simulink model "Hybrid2_article_SVC_stage1"  (R2025a)
settings: Solver=FixedStepAuto  StartTime=0.0  StopTime=0.2  FixedStep=Ts  RelTol=1e-3
undefined symbols (not defined in the file or in its folder): closedLoop, controller, D1, D11, Delta, DiscIntNeverNeededParam, find_system, grid, level, protection, sensor, solarPanel, solarPlant, Ts
libraries: powerlib_extras x38, nesl_utility x29, spsSampleandHoldLib x24, spsThyristorLib x24, spsSeriesRLCBranchLib x23, simulink x22, fl_lib x18, ee_lib x12, spsEdgeDetectorLib x12, spsParallelRLCBranchLib x10, spsThreePhaseVIMeasurementLib x9, simulink_extras x8
(part 6 of 8)

== system Hybrid2_article_SVC_stage1/Distribution Statcom1/D_statcom_avg Controller/Controller (sample time=Ts*32)/Current Regulator ==
  note: =================
  note: Current Regulators
  IdIq : Inport  PortDimensions=2
  IdIq_Ref : Inport  Port=2  PortDimensions=2
  Demux : Demux  Outputs=2
      settings: DisplayOption=none
  Demux1 : Demux  Outputs=2
      settings: DisplayOption=none
  Discrete PID Controller1 : slpidlib/PID Controller  Controller=PI  Form=Parallel  TimeDomain=Discrete-time  UseExternalTs=off  SampleTime=Ts  IntegratorMethod=Forward Euler  FilterMethod=Forward Euler  ControllerParametersSource=internal  P=Kp  I=Ki  UseKiTs=off  D=0  UseExternalDerivativeSource=off  N=100  UseFilter=on  TunerSelectOption=Transfer Function Based (PID Tuner App)  InitialConditionSource=internal  InitialConditionForIntegrator=0  InitialConditionForFilter=0  DifferentiatorICPrevScaledInput=0  ExternalReset=none  TrackingMode=off  Kt=1  LimitOutput=on  SatLimitsSource=internal  UpperSaturationLimit=1  LowerSaturationLimit=-1  LinearizeAsGain=off  AntiWindupMode=clamping  Kb=1  LimitIntegrator=off  UpperIntegratorSaturationLimit=inf  LowerIntegratorSaturationLimit=-inf  POutMin=[]  POutMax=[]  IOutMin=[]  IOutMax=[]  DOutMin=[]  DOutMax=[]  NOutMin=[]  NOutMax=[]  SumOutMin=[]  SumOutMax=[]  SaturationOutMin=[]  SaturationOutMax=[]  PParamMin=[]  PParamMax=[]  IParamMin=[]  IParamMax=[]  DParamMin=[]  DParamMax=[]  NParamMin=[]  NParamMax=[]  KbParamMin=[]  KbParamMax=[]  KtParamMin=[]  KtParamMax=[]  KbOutMin=[]  KbOutMax=[]  KtOutMin=[]  KtOutMax=[]  IntegratorOutMin=[]  IntegratorOutMax=[]  FilterOutMin=[]  FilterOutMax=[]  SumI1OutMin=[]  SumI1OutMax=[]  SumI2OutMin=[]  SumI2OutMax=[]  SumI3OutMin=[]  SumI3OutMax=[]  SumI4OutMin=[]  SumI4OutMax=[]  SumDOutMin=[]  SumDOutMax=[]  DifferentiatorOutMin=[]  DifferentiatorOutMax=[]  FilterDiffOutCoefMin=[]  FilterDiffOutCoefMax=[]  ReciprocalOutMin=[]  ReciprocalOutMax=[]  SumDenOutMin=[]  SumDenOutMax=[]  SumNumOutMin=[]  SumNumOutMax=[]  DivideOutMin=[]  DivideOutMax=[]  UdiffTsProdOutMin=[]  UdiffTsProdOutMax=[]  NTsProdOutMin=[]  NTsProdOutMax=[]  UintegralTsProdOutMin=[]  UintegralTsProdOutMax=[]  UngainTsProdOutMin=[]  UngainTsProdOutMax=[]  ClampingZeroOutDataTypeStr=Inherit: Inherit via back propagation  ClampingZeroOutMin=[]  ClampingZeroOutMax=[]  FilterDenConstantOutDataTypeStr=Inherit: Inherit via back propagation  FilterDenConstantOutMin=[]  FilterDenConstantOutMax=[]  PCopyOutDataTypeStr=Inherit: Inherit via back propagation  PCopyOutMin=[]  PCopyOutMax=[]  NCopyOutDataTypeStr=Inherit: Inherit via back propagation  NCopyOutMin=[]  NCopyOutMax=[]  IntegratorContinuousStateAttributes=''  IntegratorStateMustResolveToSignalObject=off  IntegratorRTWStateStorageClass=Auto  FilterContinuousStateAttributes=''  FilterStateMustResolveToSignalObject=off  FilterRTWStateStorageClass=Auto  ParallelPVariant=InternalParameters  IdealPVariant=Disabled  IVariant=InternalParameters  DVariant=Disabled  IntegratorVariant=Discrete  SatVariant=Enabled  AWVariant=DiscClampingParallel  PCopyVariant=Disabled  TRVariant=Disabled  FdbkBlocksVariant=Forward  IdealPFdbkVariant=Disabled  SatFdbkVariant=Disabled  DerivativeFilterVariant=Disabled  NVariant=Disabled  NCopyVariant=Disabled_SignalSpec  FilterICVariant=Disabled  IntegratorICVariant=InternalICs  ExternalResetVariant=Disabled  TRSumVariant=Passthrough  SumFdbkVariant=Disabled  SumVariant=Sum_PI  TsampFilterVariant=InternalTs  TsampNgainVariant=Passthrough  TsampIntegralVariant=Disabled_SignalSpec  ExternalSaturationOutDataTypeStr=Inherit: Same as second input  DerivativeSourceVariant=Disabled  PreIntVariant=InternalPreInt
      settings: AttributesFormatString=P = %<P>\nI = %<I>
  Discrete PID Controller2 : slpidlib/PID Controller  Controller=PI  Form=Parallel  TimeDomain=Discrete-time  UseExternalTs=off  SampleTime=Ts  IntegratorMethod=Forward Euler  FilterMethod=Forward Euler  ControllerParametersSource=internal  P=Kp  I=Ki  UseKiTs=off  D=0  UseExternalDerivativeSource=off  N=100  UseFilter=on  TunerSelectOption=Transfer Function Based (PID Tuner App)  InitialConditionSource=internal  InitialConditionForIntegrator=0  InitialConditionForFilter=0  DifferentiatorICPrevScaledInput=0  ExternalReset=none  TrackingMode=off  Kt=1  LimitOutput=on  SatLimitsSource=internal  UpperSaturationLimit=1  LowerSaturationLimit=-1  LinearizeAsGain=off  AntiWindupMode=clamping  Kb=1  LimitIntegrator=off  UpperIntegratorSaturationLimit=inf  LowerIntegratorSaturationLimit=-inf  POutMin=[]  POutMax=[]  IOutMin=[]  IOutMax=[]  DOutMin=[]  DOutMax=[]  NOutMin=[]  NOutMax=[]  SumOutMin=[]  SumOutMax=[]  SaturationOutMin=[]  SaturationOutMax=[]  PParamMin=[]  PParamMax=[]  IParamMin=[]  IParamMax=[]  DParamMin=[]  DParamMax=[]  NParamMin=[]  NParamMax=[]  KbParamMin=[]  KbParamMax=[]  KtParamMin=[]  KtParamMax=[]  KbOutMin=[]  KbOutMax=[]  KtOutMin=[]  KtOutMax=[]  IntegratorOutMin=[]  IntegratorOutMax=[]  FilterOutMin=[]  FilterOutMax=[]  SumI1OutMin=[]  SumI1OutMax=[]  SumI2OutMin=[]  SumI2OutMax=[]  SumI3OutMin=[]  SumI3OutMax=[]  SumI4OutMin=[]  SumI4OutMax=[]  SumDOutMin=[]  SumDOutMax=[]  DifferentiatorOutMin=[]  DifferentiatorOutMax=[]  FilterDiffOutCoefMin=[]  FilterDiffOutCoefMax=[]  ReciprocalOutMin=[]  ReciprocalOutMax=[]  SumDenOutMin=[]  SumDenOutMax=[]  SumNumOutMin=[]  SumNumOutMax=[]  DivideOutMin=[]  DivideOutMax=[]  UdiffTsProdOutMin=[]  UdiffTsProdOutMax=[]  NTsProdOutMin=[]  NTsProdOutMax=[]  UintegralTsProdOutMin=[]  UintegralTsProdOutMax=[]  UngainTsProdOutMin=[]  UngainTsProdOutMax=[]  ClampingZeroOutDataTypeStr=Inherit: Inherit via back propagation  ClampingZeroOutMin=[]  ClampingZeroOutMax=[]  FilterDenConstantOutDataTypeStr=Inherit: Inherit via back propagation  FilterDenConstantOutMin=[]  FilterDenConstantOutMax=[]  PCopyOutDataTypeStr=Inherit: Inherit via back propagation  PCopyOutMin=[]  PCopyOutMax=[]  NCopyOutDataTypeStr=Inherit: Inherit via back propagation  NCopyOutMin=[]  NCopyOutMax=[]  IntegratorContinuousStateAttributes=''  IntegratorStateMustResolveToSignalObject=off  IntegratorRTWStateStorageClass=Auto  FilterContinuousStateAttributes=''  FilterStateMustResolveToSignalObject=off  FilterRTWStateStorageClass=Auto  ParallelPVariant=InternalParameters  IdealPVariant=Disabled  IVariant=InternalParameters  DVariant=Disabled  IntegratorVariant=Discrete  SatVariant=Enabled  AWVariant=DiscClampingParallel  PCopyVariant=Disabled  TRVariant=Disabled  FdbkBlocksVariant=Forward  IdealPFdbkVariant=Disabled  SatFdbkVariant=Disabled  DerivativeFilterVariant=Disabled  NVariant=Disabled  NCopyVariant=Disabled_SignalSpec  FilterICVariant=Disabled  IntegratorICVariant=InternalICs  ExternalResetVariant=Disabled  TRSumVariant=Passthrough  SumFdbkVariant=Disabled  SumVariant=Sum_PI  TsampFilterVariant=InternalTs  TsampNgainVariant=Passthrough  TsampIntegralVariant=Disabled_SignalSpec  ExternalSaturationOutDataTypeStr=Inherit: Same as second input  DerivativeSourceVariant=Disabled  PreIntVariant=InternalPreInt
      settings: AttributesFormatString=P = %<P>\nI = %<I>
  Mux : Mux  Inputs=2
  Rate Limiter : RateLimiter  RisingSlewLimit=240  FallingSlewLimit=-240  SampleTimeMode=inherited
      settings: AttributesFormatString=Up = %<RisingSlewLimit>\nDown = %<FallingSlewLimit>\nIC = %<InitialCondition>
  Sum : Sum  Inputs=|+-  InputSameDT=on  SaturateOnIntegerOverflow=on  OutDataTypeStr=Inherit: Same as first input
  Sum1 : Sum  Inputs=|+-  InputSameDT=on  SaturateOnIntegerOverflow=on  OutDataTypeStr=Inherit: Same as first input
  VdVq : Outport  VectorParamsAs1DForOutWhenUnconnected=off
  wires:
  Rate Limiter/1 -> Demux1/1
  IdIq_Ref/1 -> Rate Limiter/1
  Mux/1 -> VdVq/1
  Sum/1 -> Discrete PID Controller1/1
  Demux1/2 -> Sum1/2  "Iq_Ref"
  Sum1/1 -> Discrete PID Controller2/1
  Demux/2 -> Sum1/1  "Iq"
  Demux1/1 -> Sum/2  "Id_Ref"
  Demux/1 -> Sum/1  "Id"
  IdIq/1 -> Demux/1
  Discrete PID Controller1/1 -> Mux/1  "Vd"
  Discrete PID Controller2/1 -> Mux/2  "Vq"

== system Hybrid2_article_SVC_stage1/Distribution Statcom1/D_statcom_avg Controller/Controller (sample time=Ts*32)/DC Voltage Regulator ==
  Vdc : Inport
  Vdc_Ref : Inport  Port=2
  -1<Id<+1 : Saturate  UpperLimit=1  LowerLimit=-1
  2250<Vdc<3750 : Saturate  UpperLimit=3750  LowerLimit=2250
  Discrete PI Controller : slpidlib/PID Controller  Controller=PI  Form=Parallel  TimeDomain=Discrete-time  UseExternalTs=off  SampleTime=Ts  IntegratorMethod=Forward Euler  FilterMethod=Forward Euler  ControllerParametersSource=internal  P=Kp  I=Ki  UseKiTs=off  D=0  UseExternalDerivativeSource=off  N=100  UseFilter=on  TunerSelectOption=Transfer Function Based (PID Tuner App)  InitialConditionSource=internal  InitialConditionForIntegrator=0  InitialConditionForFilter=0  DifferentiatorICPrevScaledInput=0  ExternalReset=none  TrackingMode=off  Kt=1  LimitOutput=on  SatLimitsSource=internal  UpperSaturationLimit=1  LowerSaturationLimit=-1  LinearizeAsGain=off  AntiWindupMode=clamping  Kb=1  LimitIntegrator=off  UpperIntegratorSaturationLimit=inf  LowerIntegratorSaturationLimit=-inf  POutMin=[]  POutMax=[]  IOutMin=[]  IOutMax=[]  DOutMin=[]  DOutMax=[]  NOutMin=[]  NOutMax=[]  SumOutMin=[]  SumOutMax=[]  SaturationOutMin=[]  SaturationOutMax=[]  PParamMin=[]  PParamMax=[]  IParamMin=[]  IParamMax=[]  DParamMin=[]  DParamMax=[]  NParamMin=[]  NParamMax=[]  KbParamMin=[]  KbParamMax=[]  KtParamMin=[]  KtParamMax=[]  KbOutMin=[]  KbOutMax=[]  KtOutMin=[]  KtOutMax=[]  IntegratorOutMin=[]  IntegratorOutMax=[]  FilterOutMin=[]  FilterOutMax=[]  SumI1OutMin=[]  SumI1OutMax=[]  SumI2OutMin=[]  SumI2OutMax=[]  SumI3OutMin=[]  SumI3OutMax=[]  SumI4OutMin=[]  SumI4OutMax=[]  SumDOutMin=[]  SumDOutMax=[]  DifferentiatorOutMin=[]  DifferentiatorOutMax=[]  FilterDiffOutCoefMin=[]  FilterDiffOutCoefMax=[]  ReciprocalOutMin=[]  ReciprocalOutMax=[]  SumDenOutMin=[]  SumDenOutMax=[]  SumNumOutMin=[]  SumNumOutMax=[]  DivideOutMin=[]  DivideOutMax=[]  UdiffTsProdOutMin=[]  UdiffTsProdOutMax=[]  NTsProdOutMin=[]  NTsProdOutMax=[]  UintegralTsProdOutMin=[]  UintegralTsProdOutMax=[]  UngainTsProdOutMin=[]  UngainTsProdOutMax=[]  ClampingZeroOutDataTypeStr=Inherit: Inherit via back propagation  ClampingZeroOutMin=[]  ClampingZeroOutMax=[]  FilterDenConstantOutDataTypeStr=Inherit: Inherit via back propagation  FilterDenConstantOutMin=[]  FilterDenConstantOutMax=[]  PCopyOutDataTypeStr=Inherit: Inherit via back propagation  PCopyOutMin=[]  PCopyOutMax=[]  NCopyOutDataTypeStr=Inherit: Inherit via back propagation  NCopyOutMin=[]  NCopyOutMax=[]  IntegratorContinuousStateAttributes=''  IntegratorStateMustResolveToSignalObject=off  IntegratorRTWStateStorageClass=Auto  FilterContinuousStateAttributes=''  FilterStateMustResolveToSignalObject=off  FilterRTWStateStorageClass=Auto  ParallelPVariant=InternalParameters  IdealPVariant=Disabled  IVariant=InternalParameters  DVariant=Disabled  IntegratorVariant=Discrete  SatVariant=Enabled  AWVariant=DiscClampingParallel  PCopyVariant=Disabled  TRVariant=Disabled  FdbkBlocksVariant=Forward  IdealPFdbkVariant=Disabled  SatFdbkVariant=Disabled  DerivativeFilterVariant=Disabled  NVariant=Disabled  NCopyVariant=Disabled_SignalSpec  FilterICVariant=Disabled  IntegratorICVariant=InternalICs  ExternalResetVariant=Disabled  TRSumVariant=Passthrough  SumFdbkVariant=Disabled  SumVariant=Sum_PI  TsampFilterVariant=InternalTs  TsampNgainVariant=Passthrough  TsampIntegralVariant=Disabled_SignalSpec  ExternalSaturationOutDataTypeStr=Inherit: Same as second input  DerivativeSourceVariant=Disabled  PreIntVariant=InternalPreInt
      settings: AttributesFormatString=P = %<P>\nI = %<I>
  Rate Limiter : RateLimiter  RisingSlewLimit=10000  FallingSlewLimit=-10000  SampleTimeMode=inherited  InitialCondition=3000
      settings: AttributesFormatString=Up = %<RisingSlewLimit>\nDown = %<FallingSlewLimit>\nIC = %<InitialCondition>
  Sum : Sum  Inputs=|+-  InputSameDT=on  SaturateOnIntegerOverflow=on  OutDataTypeStr=Inherit: Same as first input
  Id_Ref : Outport  InitialOutput=0  VectorParamsAs1DForOutWhenUnconnected=off
  wires:
  Vdc_Ref/1 -> 2250<Vdc<3750/1
  2250<Vdc<3750/1 -> Rate Limiter/1
  Vdc/1 -> Sum/2
  Rate Limiter/1 -> Sum/1
  -1<Id<+1/1 -> Id_Ref/1
  Sum/1 -> Discrete PI Controller/1
  Discrete PI Controller/1 -> -1<Id<+1/1

== system Hybrid2_article_SVC_stage1/Distribution Statcom1/D_statcom_avg Controller/Controller (sample time=Ts*32)/Iq_ref (Manual) ==
  MagV : Inport  PortDimensions=1
  Qref : Inport  Port=2  PortDimensions=1
  -1<Iq<+1 : Saturate  UpperLimit=1  LowerLimit=-1
  Constant11 : Constant  Value=0
  Constant13 : Constant  Value=1e-6
  Deg->Rad1 : Gain  Gain=-1  SaturateOnIntegerOverflow=on  OutDataTypeStr=Inherit: Same as input  ParamDataTypeStr=Inherit: Same as input
  Product : Product  Inputs=*/  InputSameDT=on  SaturateOnIntegerOverflow=on  OutDataTypeStr=Inherit: Same as first input
  Rate Limiter : RateLimiter  RisingSlewLimit=60*2  FallingSlewLimit=-60*2  SampleTimeMode=inherited
      settings: AttributesFormatString=Up = %<RisingSlewLimit>\nDown = %<FallingSlewLimit>
  Relational Operator1 : RelationalOperator  Operator=~=
  Second-Order Low Pass Filter : spsSecondOrderFilterLib/Second-Order Filter  FilterType=Lowpass  Fo=20  Zeta=0.707  Ts=4*Ts  Initialize=off  Vac_Init="[0,  0,  60]"  Vdc_Init=0  PlotResponse=off  FreqRange=[0, 500, 1]
      settings: AttributesFormatString=f0: %<Fo>
  Switch : Switch  Criteria=u2 > Threshold
  Iqref* : Outport  VectorParamsAs1DForOutWhenUnconnected=off
  wires:
  Rate Limiter/1 -> Product/1
  Qref/1 -> Rate Limiter/1
  -1<Iq<+1/1 -> Iqref*/1
  Deg->Rad1/1 -> -1<Iq<+1/1
  Product/1 -> Deg->Rad1/1
  Constant13/1 -> Switch/3
  MagV/1 -> Switch/1, Relational Operator1/1
  Relational Operator1/1 -> Switch/2
  Constant11/1 -> Relational Operator1/2
  Second-Order Low Pass Filter/1 -> Product/2
  Switch/1 -> Second-Order Low Pass Filter/1

== system Hybrid2_article_SVC_stage1/Distribution Statcom1/D_statcom_avg Controller/Controller (sample time=Ts*32)/Measuremnt Unit ==
  wt : Inport
  Vabc : Inport  Port=2
  Iabc : Inport  Port=3
  "Mag_V " : Fcn  Expr=sqrt(u[1]*u[1]+u[2]*u[2])
  Selector : Selector  InputPortWidth=3  IndexOptions=Index vector (dialog)  Indices=[1 2]  OutputSizes=1
  Selector1 : Selector  InputPortWidth=3  IndexOptions=Index vector (dialog)  Indices=[1 2]  OutputSizes=1
  abc to dq0 : spsabctodq0Lib/abc to dq0  Alignment=90 degrees behind phase A axis
  abc to dq1 : spsabctodq0Lib/abc to dq0  Alignment=90 degrees behind phase A axis
  IdIq : Outport  VectorParamsAs1DForOutWhenUnconnected=off
  MagV : Outport  Port=2  VectorParamsAs1DForOutWhenUnconnected=off
  tag scope: IdIq=global, VdVq=global
  wires:
  "Mag_V "/1 -> MagV/1
  Selector1/1 -> [IdIq], IdIq/1
  Selector/1 -> "Mag_V "/1, [VdVq]
  abc to dq1/1 -> Selector1/1
  Iabc/1 -> abc to dq1/1
  abc to dq0/1 -> Selector/1
  Vabc/1 -> abc to dq0/1
  wt/1 -> abc to dq1/2, abc to dq0/2

== system Hybrid2_article_SVC_stage1/Distribution Statcom1/D_statcom_avg Controller/Controller (sample time=Ts*32)/Vd_Vq--> m,Phi ==
  VdVq : Inport
  Fcn3 : Fcn  Expr=sqrt(u[1]*u[1]+u[2]*u[2])
  Fcn4 : Fcn  Expr=atan2(u[2]+1e-6,u[1])*180/pi
  Mux2 : Mux  Inputs=2
  m_Phi : Outport  VectorParamsAs1DForOutWhenUnconnected=off
  wires:
  Fcn4/1 -> Mux2/2
  Mux2/1 -> m_Phi/1
  Fcn3/1 -> Mux2/1
  VdVq/1 -> Fcn4/1, Fcn3/1

== system Hybrid2_article_SVC_stage1/MPPT/MPPT Algorithm/IncrementalConductance/If Action Subsystem ==
  delI : Inport
  Action Port : ActionPort  ActionPortLabel=if(u1 == 0)
  Compare To Constant : simulink/Logic and Bit Operations/Compare To Constant  relop===  const=0  OutDataTypeStr=boolean
  Compare To Zero2 : simulink/Logic and Bit Operations/Compare To Zero  relop=>  OutDataTypeStr=boolean
  Set : Outport  VectorParamsAs1DForOutWhenUnconnected=off
  Inc : Outport  Port=2  VectorParamsAs1DForOutWhenUnconnected=off
  wires:
  Compare To Constant/1 -> Set/1  "Yes"
  Compare To Zero2/1 -> Inc/1  "Yes"
  delI/1 -> Compare To Zero2/1, Compare To Constant/1  "delI"

== system Hybrid2_article_SVC_stage1/MPPT/MPPT Algorithm/IncrementalConductance/If Action Subsystem1 ==
  delI : Inport
  delV : Inport  Port=2
  Vpv : Inport  Port=3
  Ipv : Inport  Port=4
  Action Port : ActionPort  ActionPortLabel=else
  Add : Sum
  Compare To Zero : simulink/Logic and Bit Operations/Compare To Zero  relop===  OutDataTypeStr=boolean
  Compare To Zero1 : simulink/Logic and Bit Operations/Compare To Zero  relop=>  OutDataTypeStr=boolean
  Divide : Product  Inputs=*/
  Product : Product
  Set : Outport  VectorParamsAs1DForOutWhenUnconnected=off
  Inc : Outport  Port=2  VectorParamsAs1DForOutWhenUnconnected=off
  wires:
  delI/1 -> Divide/1
  delV/1 -> Divide/2
  Divide/1 -> Product/1
  Add/1 -> Compare To Zero1/1, Compare To Zero/1
  Compare To Zero1/1 -> Inc/1  "increase"
  Compare To Zero/1 -> Set/1  "set"
  Vpv/1 -> Product/2
  Product/1 -> Add/1
  Ipv/1 -> Add/2

== system Hybrid2_article_SVC_stage1/Power Circuit/Power Circuit/Three Level/Gate ==
  g : Inport
  Demux : Demux  Outputs=12
  Simulink-PS Converter{,1..11} (12 alike) : nesl_utility/Simulink-PS Converter  PhysicalDomain=network_engine_domain  SubClassName=ps_input  LeftPortType=input  RightPortType=output  PseudoPeriodic=off  Frequencies=[]  NoiseDistribution=none  NoiseParameters=[]  Unit=1  AffineConversion=off  FilteringAndDerivatives=zero  SimscapeFilterOrder=1  InputFilterTimeConstant=0.001  UdotUserProvided=1
  Twelve-Pulse Gate Multiplexer : ee_lib/Semiconductors & Converters/Converters/Twelve-Pulse Gate Multiplexer  port_option=ee.enum.controlport.ps
      settings: InternalSimscapePortConfiguration="{\"Bottom\":[],\"Left\":[{\"id\":\"Ga1_ps\",\"label\":\"Ga(1)\",\"type\":\"input\"},{\"id\":\"Ga2_ps\",\"label\":\"Ga(2)\",\"type\":\"input\"},{\"id\":\"Ga3_ps\",\"label\":\"Ga(3)\",\"type\":\"input\"},{\"id\":\"Ga4_ps\",\"label\":\"Ga(4)\",\"type\":\"input\"},{\"id\":\"Gb1_ps\",\"label\":\"Gb(1)\",\"type\":\"input\"},{\"id\":\"Gb2_ps\",\"label\":\"Gb(2)\",\"type\":\"input\"},{\"id\":\"Gb3_ps\",\"label\":\"Gb(3)\",\"type\":\"input\"},{\"id\":\"Gb4_ps\",\"label\":\"Gb(4)\",\"type\":\"input\"},{\"id\":\"Gc1_ps\",\"label\":\"Gc(1)\",\"type\":\"input\"},{\"id\":\"Gc2_ps\",\"label\":\"Gc(2)\",\"type\":\"input\"},{\"id\":\"Gc3_ps\",\"label\":\"Gc(3)\",\"type\":\"input\"},{\"id\":\"Gc4_ps\",\"label\":\"Gc(4)\",\"type\":\"input\"}],\"Right\":[{\"id\":\"p\",\"label\":\"G\",\"type\":\"foundation.electrical.twenty_four_phase\"}],\"Top\":[]}"
  G : PMIOPort  Side=Right
  wires:
  g/1 -> Demux/1
  Demux/5 -> Simulink-PS Converter4/1
  Demux/10 -> Simulink-PS Converter9/1
  Demux/2 -> Simulink-PS Converter1/1
  Demux/9 -> Simulink-PS Converter8/1
  Demux/12 -> Simulink-PS Converter11/1
  Demux/3 -> Simulink-PS Converter2/1
  Demux/7 -> Simulink-PS Converter6/1
  Demux/6 -> Simulink-PS Converter5/1
  Demux/4 -> Simulink-PS Converter3/1
  Demux/1 -> Simulink-PS Converter/1
  Demux/11 -> Simulink-PS Converter10/1
  Demux/8 -> Simulink-PS Converter7/1
  connections:
  Simulink-PS Converter10/RConn1 -- Twelve-Pulse Gate Multiplexer/LConn11
  Simulink-PS Converter8/RConn1 -- Twelve-Pulse Gate Multiplexer/LConn9
  Simulink-PS Converter/RConn1 -- Twelve-Pulse Gate Multiplexer/LConn1
  Simulink-PS Converter11/RConn1 -- Twelve-Pulse Gate Multiplexer/LConn12
  Simulink-PS Converter3/RConn1 -- Twelve-Pulse Gate Multiplexer/LConn4
  Simulink-PS Converter2/RConn1 -- Twelve-Pulse Gate Multiplexer/LConn3
  Simulink-PS Converter4/RConn1 -- Twelve-Pulse Gate Multiplexer/LConn5
  Simulink-PS Converter1/RConn1 -- Twelve-Pulse Gate Multiplexer/LConn2
  Twelve-Pulse Gate Multiplexer/RConn1 -- G/RConn1
  Simulink-PS Converter5/RConn1 -- Twelve-Pulse Gate Multiplexer/LConn6
  Simulink-PS Converter9/RConn1 -- Twelve-Pulse Gate Multiplexer/LConn10
  Simulink-PS Converter6/RConn1 -- Twelve-Pulse Gate Multiplexer/LConn7
  Simulink-PS Converter7/RConn1 -- Twelve-Pulse Gate Multiplexer/LConn8

== system Hybrid2_article_SVC_stage1/Power Circuit/Power Circuit/Three Level/Protection ==
  TripSig : Inport
  G : Inport  Port=2
  Constant2 : Constant  Value=0
  NOT : Logic  Operator=NOT  IconShape=distinctive  AllPortsSameDT=off  OutDataTypeStr=boolean
  Switch : Switch  Criteria=u2 > Threshold  SaturateOnIntegerOverflow=off  InputSameDT=off
  PWM : Outport  VectorParamsAs1DForOutWhenUnconnected=off
  wires:
  NOT/1 -> Switch/2
  Constant2/1 -> Switch/3
  Switch/1 -> PWM/1
  G/1 -> Switch/1
  TripSig/1 -> NOT/1

== system Hybrid2_article_SVC_stage1/Power Circuit/Power Circuit/Three Level/Sensing voltage Vc1 ==
  PS-Simulink Converter : nesl_utility/PS-Simulink Converter  PhysicalDomain=network_engine_domain  SubClassName=ps_output  LeftPortType=input  RightPortType=output  PseudoPeriodic=off  Frequencies=[]  VectorFormat=1-D array  Unit=1  AffineConversion=off
  Sensor dynamics : TransferFcn  Numerator=1  Denominator=[1/sensor.samplingFreq 1]
  Vc1 : fl_lib/Electrical/Electrical Sensors/Voltage Sensor
  + : PMIOPort  Side=Left
  - : PMIOPort  Port=2  Side=Right
  tag scope: Vdc1=global
  wires:
  PS-Simulink Converter/1 -> Sensor dynamics/1
  Sensor dynamics/1 -> [Vdc1]
  connections:
  Vc1/RConn2 -- -/RConn1
  Vc1/LConn1 -- +/RConn1
  PS-Simulink Converter/LConn1 -- Vc1/RConn1

== system Hybrid2_article_SVC_stage1/Power Circuit/Power Circuit/Three Level/Sensing voltage Vc2 ==
  PS-Simulink Converter : nesl_utility/PS-Simulink Converter  PhysicalDomain=network_engine_domain  SubClassName=ps_output  LeftPortType=input  RightPortType=output  PseudoPeriodic=off  Frequencies=[]  VectorFormat=1-D array  Unit=1  AffineConversion=off
  Sensor dynamics : TransferFcn  Numerator=1  Denominator=[1/sensor.samplingFreq 1]
  Vc2 : fl_lib/Electrical/Electrical Sensors/Voltage Sensor
  Conn1 : PMIOPort  Side=Left
  Conn3 : PMIOPort  Port=2  Side=Right
  tag scope: Vdc2=global
  wires:
  Sensor dynamics/1 -> [Vdc2]
  PS-Simulink Converter/1 -> Sensor dynamics/1
  connections:
  Vc2/RConn2 -- Conn3/RConn1
  Vc2/LConn1 -- Conn1/RConn1
  PS-Simulink Converter/LConn1 -- Vc2/RConn1

== system Hybrid2_article_SVC_stage1/Power Circuit/Power Circuit/Two Level/Protection ==
  G : Inport
  TripSig : Inport  Port=2
  Constant : Constant  Value=5
  Constant2 : Constant  Value=0
  NOT : Logic  Operator=NOT  IconShape=distinctive  AllPortsSameDT=off  OutDataTypeStr=boolean
  Subtract : Sum  Inputs=-+
  Switch : Switch  Criteria=u2 > Threshold  SaturateOnIntegerOverflow=off  InputSameDT=off
  Switch1 : Switch  Criteria=u2 > Threshold  SaturateOnIntegerOverflow=off  InputSameDT=off
  G1 : Outport  VectorParamsAs1DForOutWhenUnconnected=off
  G2 : Outport  Port=2  VectorParamsAs1DForOutWhenUnconnected=off
  wires:
  Switch1/1 -> G2/1
  NOT/1 -> Switch/2
  Constant2/1 -> Switch/3, Switch1/1
  Constant/1 -> Subtract/2
  Switch/1 -> G1/1
  Subtract/1 -> Switch1/3
  G/1 -> Switch/1, Subtract/1
  TripSig/1 -> Switch1/2, NOT/1

== system Hybrid2_article_SVC_stage1/SVC Controller1/Firing Unit/Firing Unit AB/BL2 ==
  Freq : Inport  PortDimensions=1
  Constant1 : Constant  Value=0
  Constant2 : Constant  Value=1e-5
  Constant3 : Constant
  Gain : Gain  Gain=Ts  SaturateOnIntegerOverflow=on  OutDataTypeStr=Inherit: Same as input  ParamDataTypeStr=Inherit: Same as input
  Product : Product  Inputs=/*  InputSameDT=on  SaturateOnIntegerOverflow=on  OutDataTypeStr=Inherit: Same as first input
  Relational Operator1 : RelationalOperator  Operator=~=
  Switch : Switch  Threshold=0.5
  Ns/c : Outport  VectorParamsAs1DForOutWhenUnconnected=off
  wires:
  Product/1 -> Ns/c/1
  Freq/1 -> Gain/1
  Constant1/1 -> Relational Operator1/2
  Gain/1 -> Relational Operator1/1, Switch/1
  Constant2/1 -> Switch/3
  Relational Operator1/1 -> Switch/2
  Switch/1 -> Product/1
  Constant3/1 -> Product/2

== system Hybrid2_article_SVC_stage1/SVC Controller1/Firing Unit/Firing Unit AB/BL3 ==
  Freq : Inport  PortDimensions=1
  sin(wt) : Inport  Port=2  PortDimensions=1
  Bistable : spsBistableLib/Bistable  Qpriority=Set  ic=0  Ts=Ts
  Data Type Conversion : DataTypeConversion  SaturateOnIntegerOverflow=off  RndMeth=Floor
  Edge Detector : spsEdgeDetectorLib/Edge Detector  model=Rising  ic=0  Ts=Ts
  Edge Detector1 : spsEdgeDetectorLib/Edge Detector  model=Falling  ic=0  Ts=Ts
  Edge Detector2 : spsEdgeDetectorLib/Edge Detector  model=Rising  ic=0  Ts=Ts
  Edge Detector3 : spsEdgeDetectorLib/Edge Detector  model=Rising  ic=0  Ts=Ts
  Product2 : Product  InputSameDT=on  SaturateOnIntegerOverflow=on  OutDataTypeStr=Inherit: Same as first input
  Relational Operator : RelationalOperator  Operator=>
  Relational Operator2 : RelationalOperator  Operator=<
  Sum5 : Sum  Inputs=+-  InputSameDT=on  SaturateOnIntegerOverflow=on  OutDataTypeStr=Inherit: Same as first input
  Sum6 : Sum  InputSameDT=on  SaturateOnIntegerOverflow=on  OutDataTypeStr=Inherit: Same as first input
  Terminator : Terminator
  Trigonometric Function7 : Trigonometry
  alpha2 : Constant  Value=0
  alpha9 : Constant  Value=pi*Ts
  SqWave : Outport  VectorParamsAs1DForOutWhenUnconnected=off
  Sync + : Outport  Port=2  VectorParamsAs1DForOutWhenUnconnected=off
  Sync - : Outport  Port=3  VectorParamsAs1DForOutWhenUnconnected=off
  wires:
  Data Type Conversion/1 -> Edge Detector/1, Edge Detector1/1, SqWave/1
  Bistable/2 -> Terminator/1
  Edge Detector3/1 -> Bistable/2
  Edge Detector2/1 -> Bistable/1
  Edge Detector1/1 -> Sync -/1
  Edge Detector/1 -> Sync +/1
  Bistable/1 -> Data Type Conversion/1
  alpha9/1 -> Product2/1
  Product2/1 -> Trigonometric Function7/1
  Relational Operator2/1 -> Edge Detector3/1
  Relational Operator/1 -> Edge Detector2/1
  Sum6/1 -> Relational Operator2/2
  Sum5/1 -> Relational Operator/2
  alpha2/1 -> Sum6/1, Sum5/1
  Trigonometric Function7/1 -> Sum6/2, Sum5/2
  Freq/1 -> Product2/2
  sin(wt)/1 -> Relational Operator/1, Relational Operator2/1

== system Hybrid2_article_SVC_stage1/SVC Controller1/Firing Unit/Firing Unit AB/PLL sync on positive peak  ==
  note: Note: -sin( a ) * sin( b ) = 1/2 * cos( a+b ) - 1/2 * cos(a-b)
  note: Discrete 1-phase PLL
  note: Note: PLL synchronized on positive peak of input
  note: Pierre Giroux, Gilbert Sybille
      | Power System Laboratory, IREQ
      | Hydro-Quebec
  V(pu) : Inport
  Constant4 : Constant  Value=2*pi
  Discrete PI Controller : Subsystem  DialogController=POWERSYS.PowerSysDialog  mask(Discrete PI Controller){Kp=Kp, Ki=Ki, Par_Limits=[1.25  0.75]*2*pi*Finit, Init=2*pi*Finit, Ts=Ts}
      mask prompts: Kp "Proportional gain (Kp):"; Ki "Integral gain (Ki):"; Par_Limits "Output limits: [ Upper   Lower ]"; Init "Output initial value:"; Ts "Sample time:"
      mask help: This block implements a discrete PI controller.
      mask init:
      | UpperLimit=Par_Limits(1);
      | LowerLimit=Par_Limits(2);
      | power_initmask();
      mask Help: This block is part of a subset of blocks in the Extras library that does not have documentation associated with it, other than the block mask description.
      mask Display: disp('PI');
  Discrete-Time Integrator : DiscreteIntegrator  InitialCondition=(Phase_Init-90)*pi/180  SampleTime=Ts  ICPrevOutput=DiscIntNeverNeededParam  ICPrevScaledInput=DiscIntNeverNeededParam
  Gain10 : Gain  Gain=1/2/pi  SaturateOnIntegerOverflow=on  OutDataTypeStr=Inherit: Same as input  ParamDataTypeStr=Inherit: Same as input
  Gain12 : Gain  Gain=-1  SaturateOnIntegerOverflow=on  OutDataTypeStr=Inherit: Same as input  ParamDataTypeStr=Inherit: Same as input
  Math Function : Math  Operator=mod  SignedPower=on
  Mean (Variable Frequency)1 : spsMeanVariableFrequencyLib/Mean (Variable Frequency)  Finit=Finit  Fmin=45  Vinit=0  Ts=Ts
  Product1 : Product  InputSameDT=on  SaturateOnIntegerOverflow=on  OutDataTypeStr=Inherit: Same as first input
  Rate Limiter : RateLimiter  RisingSlewLimit=10  FallingSlewLimit=-10  SampleTimeMode=inherited  InitialCondition=Finit
  Second-Order Filter : spsSecondOrderFilterLib/Second-Order Filter  FilterType=Lowpass  Fo=25  Zeta=0.707  Ts=Ts  Initialize=on  Vac_Init="[0 0  Finit]"  Vdc_Init=Finit  PlotResponse=off  FreqRange=[1 500 1]
  Trigonometric Function6 : Trigonometry
  Unit Delay1 : UnitDelay  InitialCondition=Finit  SampleTime=Ts  HasFrameUpgradeWarning=on
      settings: AttributesFormatString=IC = %<InitialCondition>
  Freq : Outport  VectorParamsAs1DForOutWhenUnconnected=off
  wt : Outport  Port=2  VectorParamsAs1DForOutWhenUnconnected=off
  wires:
  Gain12/1 -> Product1/1
  V(pu)/1 -> Gain12/1
  Constant4/1 -> Math Function/2
  Discrete-Time Integrator/1 -> Math Function/1
  Product1/1 -> Mean (Variable Frequency)1/2
  Discrete PI Controller/1(Out) -> Discrete-Time Integrator/1, Gain10/1  "W"
  Gain10/1 -> Rate Limiter/1
  Rate Limiter/1 -> Second-Order Filter/1
  Second-Order Filter/1 -> Unit Delay1/1
  Trigonometric Function6/1 -> Product1/2
  Math Function/1 -> Trigonometric Function6/1, wt/1
  Unit Delay1/1 -> Mean (Variable Frequency)1/1, Freq/1
  Mean (Variable Frequency)1/1 -> Discrete PI Controller/1(Error)

== system Hybrid2_article_SVC_stage1/SVC Controller1/Firing Unit/Firing Unit AB/TCR Pulse Generatorr ==
  Ns/c : Inport
  Alpha : Inport  Port=2  PortDimensions=1
  Sync +/- : Inport  Port=3  PortDimensions=1
  SqWave : Inport  Port=4  PortDimensions=1
  Alpha 90<A<181 : Constant  Value=90
  Alpha 90<A<182 : Constant  Value=360
  Alpha 90<A<183 : Constant  Value=2
  Alpha 90<A<184 : Constant  Value=2
  Alpha 90<A<185 : Constant  Value=87
  Data Type Conversion : DataTypeConversion  OutDataTypeStr=double  SaturateOnIntegerOverflow=off  RndMeth=Floor
  Discrete-Time Integrator : DiscreteIntegrator  ExternalReset=rising  SampleTime=Ts  LimitOutput=on  UpperSaturationLimit=100000  LowerSaturationLimit=0  ICPrevOutput=DiscIntNeverNeededParam  ICPrevScaledInput=DiscIntNeverNeededParam
  Gain2 : Gain  Gain=1/Ts  OutDataTypeStr=double  SaturateOnIntegerOverflow=on  ParamDataTypeStr=Inherit: Same as input
  Logical Operator1 : Logic  Inputs=3
  Logical Operator2 : Logic  Operator=NOT  Inputs=3
  Product : Product  Inputs=*/  InputSameDT=on  SaturateOnIntegerOverflow=on  OutDataTypeStr=Inherit: Same as first input
  Product1 : Product  Inputs=**  InputSameDT=on  SaturateOnIntegerOverflow=on  OutDataTypeStr=Inherit: Same as first input
  Product2 : Product  Inputs=*/  InputSameDT=on  SaturateOnIntegerOverflow=on  OutDataTypeStr=Inherit: Same as first input
  Relational Operator1 : RelationalOperator  Operator=<=
  Relational Operator2 : RelationalOperator
  Relational Operator3 : RelationalOperator  Operator=<=
  Rounding Function1 : Rounding  Operator=round
  Rounding Function3 : Rounding  Operator=round
  Sample and Hold : spsSampleandHoldLib/Sample and Hold  ic=180  Ts=Ts
      settings: AttributesFormatString=IC = %<ic>
  Sum1 : Sum  Inputs=+-  InputSameDT=on  SaturateOnIntegerOverflow=on  OutDataTypeStr=Inherit: Same as first input
  Sum2 : Sum  Inputs=+--  InputSameDT=on  SaturateOnIntegerOverflow=on  OutDataTypeStr=Inherit: Same as first input
  Switch : Switch  Criteria=u2 > Threshold
  TCR +/- : Outport  VectorParamsAs1DForOutWhenUnconnected=off
  wires:
  Alpha 90<A<181/1 -> Sum1/2
  Ns/c/1 -> Product1/1, Product2/1
  Product1/1 -> Rounding Function1/1
  Alpha 90<A<182/1 -> Product/2
  Product/1 -> Product1/2
  Product2/1 -> Rounding Function3/1
  Alpha 90<A<183/1 -> Product2/2
  Sum1/1 -> Product/1, Relational Operator1/1
  Alpha 90<A<185/1 -> Relational Operator1/2
  Alpha/1 -> Sample and Hold/1
  Rounding Function1/1 -> Sum2/3, Switch/1
  Rounding Function3/1 -> Sum2/1, Switch/3
  Alpha 90<A<184/1 -> Sum2/2
  Relational Operator1/1 -> Switch/2
  Relational Operator3/1 -> Logical Operator1/3
  Discrete-Time Integrator/1 -> Relational Operator2/1, Relational Operator3/1
  Relational Operator2/1 -> Logical Operator1/2
  Logical Operator1/1 -> TCR +/-/1
  Gain2/1 -> Discrete-Time Integrator/1
  Switch/1 -> Relational Operator2/2
  Sum2/1 -> Relational Operator3/2
  Logical Operator2/1 -> Discrete-Time Integrator/2
  SqWave/1 -> Data Type Conversion/1, Logical Operator1/1, Logical Operator2/1
  Sync +/-/1 -> Sample and Hold/2
  Sample and Hold/1 -> Sum1/1
  Data Type Conversion/1 -> Gain2/1

== system Hybrid2_article_SVC_stage1/SVC Controller1/Firing Unit/Firing Unit AB/TCR Pulse Generatorr1 ==
  Ns/c : Inport
  Alpha : Inport  Port=2  PortDimensions=1
  Sync +/- : Inport  Port=3  PortDimensions=1
  SqWave : Inport  Port=4  PortDimensions=1
  Alpha 90<A<181 : Constant  Value=90
  Alpha 90<A<182 : Constant  Value=360
  Alpha 90<A<183 : Constant  Value=2
  Alpha 90<A<184 : Constant  Value=2
  Alpha 90<A<185 : Constant  Value=87
  Data Type Conversion : DataTypeConversion  OutDataTypeStr=double  SaturateOnIntegerOverflow=off  RndMeth=Floor
  Discrete-Time Integrator : DiscreteIntegrator  ExternalReset=rising  SampleTime=Ts  OutDataTypeStr=double  LimitOutput=on  UpperSaturationLimit=10  LowerSaturationLimit=0  ICPrevOutput=DiscIntNeverNeededParam  ICPrevScaledInput=DiscIntNeverNeededParam
  Gain2 : Gain  Gain=1/Ts  OutDataTypeStr=double  SaturateOnIntegerOverflow=on  ParamDataTypeStr=Inherit: Same as input
  Logical Operator1 : Logic  Inputs=3
  Logical Operator2 : Logic  Operator=NOT  Inputs=3
  Product : Product  Inputs=*/  InputSameDT=on  SaturateOnIntegerOverflow=on  OutDataTypeStr=Inherit: Same as first input
  Product1 : Product  Inputs=**  InputSameDT=on  SaturateOnIntegerOverflow=on  OutDataTypeStr=Inherit: Same as first input
  Product2 : Product  Inputs=*/  InputSameDT=on  SaturateOnIntegerOverflow=on  OutDataTypeStr=Inherit: Same as first input
  Relational Operator1 : RelationalOperator  Operator=<=
  Relational Operator2 : RelationalOperator
  Relational Operator3 : RelationalOperator  Operator=<=
  Rounding Function1 : Rounding  Operator=round
  Rounding Function3 : Rounding  Operator=round
  Sample and Hold : spsSampleandHoldLib/Sample and Hold  ic=180  Ts=Ts
      settings: AttributesFormatString=IC = %<ic>
  Sum1 : Sum  Inputs=+-  InputSameDT=on  SaturateOnIntegerOverflow=on  OutDataTypeStr=Inherit: Same as first input
  Sum2 : Sum  Inputs=+--  OutDataTypeStr=Inherit: Inherit via back propagation  InputSameDT=on  SaturateOnIntegerOverflow=on
  Switch : Switch  Criteria=u2 > Threshold  OutDataTypeStr=Inherit: Inherit via back propagation  InputSameDT=off
      settings: LockScale=on
  TCR +/- : Outport  VectorParamsAs1DForOutWhenUnconnected=off
  wires:
  Alpha 90<A<181/1 -> Sum1/2
  Ns/c/1 -> Product1/1, Product2/1
  Product1/1 -> Rounding Function1/1
  Alpha 90<A<182/1 -> Product/2
  Product/1 -> Product1/2
  Product2/1 -> Rounding Function3/1
  Alpha 90<A<183/1 -> Product2/2
  Sum1/1 -> Product/1, Relational Operator1/1
  Alpha 90<A<185/1 -> Relational Operator1/2
  Alpha/1 -> Sample and Hold/1
  Rounding Function1/1 -> Sum2/3, Switch/1
  Rounding Function3/1 -> Sum2/1, Switch/3
  Alpha 90<A<184/1 -> Sum2/2
  Relational Operator1/1 -> Switch/2
  Relational Operator3/1 -> Logical Operator1/3
  Discrete-Time Integrator/1 -> Relational Operator2/1, Relational Operator3/1
  Relational Operator2/1 -> Logical Operator1/2
  Logical Operator1/1 -> TCR +/-/1
  Gain2/1 -> Discrete-Time Integrator/1
  Switch/1 -> Relational Operator2/2
  Sum2/1 -> Relational Operator3/2
  Logical Operator2/1 -> Discrete-Time Integrator/2
  SqWave/1 -> Data Type Conversion/1, Logical Operator1/1, Logical Operator2/1
  Sync +/-/1 -> Sample and Hold/2
  Sample and Hold/1 -> Sum1/1
  Data Type Conversion/1 -> Gain2/1

== system Hybrid2_article_SVC_stage1/SVC Controller1/Firing Unit/Firing Unit AB/TCS Pulse Generator ==
  note: Note: Sync+ , Sync - and SqWave signals are inverted for TSC firing (i.e. positive thyristor is fired on negative peak voltage)
  SqWave : Inport  PortDimensions=1
  Sync + : Inport  Port=2  PortDimensions=1
  Sync - : Inport  Port=3  PortDimensions=1
  TSC_On : Inport  Port=4  PortDimensions=1
  Alpha1 : Constant  Value=FiringMode-1  OutDataTypeStr=Inherit: Inherit via back propagation
  Delay : Delay  DelayLength=fix(1/FreqInit/Ts)
  Logical Operator1 : Logic  Operator=NOT
  Logical Operator10 : Logic  Operator=OR
  Logical Operator11 : Logic  Inputs=3
  Logical Operator12 : Logic
  Logical Operator13 : Logic
  Logical Operator14 : Logic  Operator=OR
  Logical Operator15 : Logic  Inputs=3
  Sample and Hold : spsSampleandHoldLib/Sample and Hold  ic=0  Ts=Ts
      settings: AttributesFormatString=IC = %<ic>
  Sample and Hold1 : spsSampleandHoldLib/Sample and Hold  ic=0  Ts=Ts
      settings: AttributesFormatString=IC = %<ic>
  TSC + : Outport  VectorParamsAs1DForOutWhenUnconnected=off
  TSC - : Outport  Port=2  VectorParamsAs1DForOutWhenUnconnected=off
  wires:
  Delay/1 -> Logical Operator14/2, Logical Operator10/2
  Logical Operator15/1 -> TSC -/1
  Logical Operator11/1 -> TSC +/1
  Logical Operator14/1 -> Logical Operator15/2
  Logical Operator10/1 -> Logical Operator11/2
  Logical Operator1/1 -> Logical Operator10/1
  SqWave/1 -> Logical Operator14/1, Logical Operator1/1
  Logical Operator12/1 -> Delay/1
  Alpha1/1 -> Logical Operator12/2
  Logical Operator13/1 -> Logical Operator12/1
  TSC_On/1 -> Sample and Hold1/1, Sample and Hold/1, Logical Operator15/3, Logical Operator11/3
  Sync -/1 -> Sample and Hold/2
  Sync +/1 -> Sample and Hold1/2
  Sample and Hold/1 -> Logical Operator13/1, Logical Operator11/1
  Sample and Hold1/1 -> Logical Operator13/2, Logical Operator15/1

== system Hybrid2_article_SVC_stage1/SVC Controller1/Firing Unit/Firing Unit AB/TCS Pulse Generator1 ==
  note: Note: Sync+ , Sync - and SqWave signals are inverted for TSC firing (i.e. positive thyristor is fired on negative peak voltage)
  SqWave : Inport  PortDimensions=1
  Sync + : Inport  Port=2  PortDimensions=1
  Sync - : Inport  Port=3  PortDimensions=1
  TSC_On : Inport  Port=4  PortDimensions=1
  Alpha1 : Constant  Value=FiringMode-1  OutDataTypeStr=boolean  LockScale=on
  Delay : Delay  DelayLength=fix(1/FreqInit/Ts)
  Logical Operator1 : Logic  Operator=NOT
  Logical Operator10 : Logic  Operator=OR
  Logical Operator11 : Logic  Inputs=3
  Logical Operator12 : Logic
  Logical Operator13 : Logic
  Logical Operator14 : Logic  Operator=OR
  Logical Operator15 : Logic  Inputs=3
  Sample and Hold : spsSampleandHoldLib/Sample and Hold  ic=0  Ts=Ts
      settings: AttributesFormatString=IC = %<ic>
  Sample and Hold1 : spsSampleandHoldLib/Sample and Hold  ic=0  Ts=Ts
      settings: AttributesFormatString=IC = %<ic>
  TSC + : Outport  VectorParamsAs1DForOutWhenUnconnected=off
  TSC - : Outport  Port=2  VectorParamsAs1DForOutWhenUnconnected=off
  wires:
  Delay/1 -> Logical Operator14/2, Logical Operator10/2
  Logical Operator15/1 -> TSC -/1
  Logical Operator11/1 -> TSC +/1
  Logical Operator14/1 -> Logical Operator15/2
  Logical Operator10/1 -> Logical Operator11/2
  Logical Operator1/1 -> Logical Operator10/1
  SqWave/1 -> Logical Operator14/1, Logical Operator1/1
  Logical Operator12/1 -> Delay/1
  Alpha1/1 -> Logical Operator12/2
  Logical Operator13/1 -> Logical Operator12/1
  TSC_On/1 -> Sample and Hold1/1, Sample and Hold/1, Logical Operator15/3, Logical Operator11/3
  Sync -/1 -> Sample and Hold/2
  Sync +/1 -> Sample and Hold1/2
  Sample and Hold/1 -> Logical Operator13/1, Logical Operator11/1
  Sample and Hold1/1 -> Logical Operator13/2, Logical Operator15/1

== system Hybrid2_article_SVC_stage1/SVC Controller1/Firing Unit/Firing Unit AB/TCS Pulse Generator2 ==
  note: Note: Sync+ , Sync - and SqWave signals are inverted for TSC firing (i.e. positive thyristor is fired on negative peak voltage)
  SqWave : Inport  PortDimensions=1
  Sync + : Inport  Port=2  PortDimensions=1
  Sync - : Inport  Port=3  PortDimensions=1
  TSC_On : Inport  Port=4  PortDimensions=1
  Alpha1 : Constant  Value=FiringMode-1  OutDataTypeStr=boolean  LockScale=on
  Delay : Delay  DelayLength=fix(1/FreqInit/Ts)
  Logical Operator1 : Logic  Operator=NOT
  Logical Operator10 : Logic  Operator=OR
  Logical Operator11 : Logic  Inputs=3
  Logical Operator12 : Logic
  Logical Operator13 : Logic
  Logical Operator14 : Logic  Operator=OR
  Logical Operator15 : Logic  Inputs=3
  Sample and Hold : spsSampleandHoldLib/Sample and Hold  ic=0  Ts=Ts
      settings: AttributesFormatString=IC = %<ic>
  Sample and Hold1 : spsSampleandHoldLib/Sample and Hold  ic=0  Ts=Ts
      settings: AttributesFormatString=IC = %<ic>
  TSC + : Outport  VectorParamsAs1DForOutWhenUnconnected=off
  TSC - : Outport  Port=2  VectorParamsAs1DForOutWhenUnconnected=off
  wires:
  Delay/1 -> Logical Operator14/2, Logical Operator10/2
  Logical Operator15/1 -> TSC -/1
  Logical Operator11/1 -> TSC +/1
  Logical Operator14/1 -> Logical Operator15/2
  Logical Operator10/1 -> Logical Operator11/2
  Logical Operator1/1 -> Logical Operator10/1
  SqWave/1 -> Logical Operator14/1, Logical Operator1/1
  Logical Operator12/1 -> Delay/1
  Alpha1/1 -> Logical Operator12/2
  Logical Operator13/1 -> Logical Operator12/1
  TSC_On/1 -> Sample and Hold1/1, Sample and Hold/1, Logical Operator15/3, Logical Operator11/3
  Sync -/1 -> Sample and Hold/2
  Sync +/1 -> Sample and Hold1/2
  Sample and Hold/1 -> Logical Operator13/1, Logical Operator11/1
  Sample and Hold1/1 -> Logical Operator13/2, Logical Operator15/1

== system Hybrid2_article_SVC_stage1/SVC Controller1/Firing Unit/Firing Unit BC/BL2 ==
  Freq : Inport  PortDimensions=1
  Constant1 : Constant  Value=0
  Constant2 : Constant  Value=1e-5
  Constant3 : Constant
  Gain : Gain  Gain=Ts  SaturateOnIntegerOverflow=on  OutDataTypeStr=Inherit: Same as input  ParamDataTypeStr=Inherit: Same as input
  Product : Product  Inputs=/*  InputSameDT=on  SaturateOnIntegerOverflow=on  OutDataTypeStr=Inherit: Same as first input
  Relational Operator1 : RelationalOperator  Operator=~=
  Switch : Switch  Threshold=0.5
  Ns/c : Outport  VectorParamsAs1DForOutWhenUnconnected=off
  wires:
  Product/1 -> Ns/c/1
  Freq/1 -> Gain/1
  Constant1/1 -> Relational Operator1/2
  Gain/1 -> Relational Operator1/1, Switch/1
  Constant2/1 -> Switch/3
  Relational Operator1/1 -> Switch/2
  Switch/1 -> Product/1
  Constant3/1 -> Product/2

== system Hybrid2_article_SVC_stage1/SVC Controller1/Firing Unit/Firing Unit BC/BL3 ==
  Freq : Inport  PortDimensions=1
  sin(wt) : Inport  Port=2  PortDimensions=1
  Bistable : spsBistableLib/Bistable  Qpriority=Set  ic=0  Ts=Ts
  Data Type Conversion : DataTypeConversion  SaturateOnIntegerOverflow=off  RndMeth=Floor
  Edge Detector : spsEdgeDetectorLib/Edge Detector  model=Rising  ic=0  Ts=Ts
  Edge Detector1 : spsEdgeDetectorLib/Edge Detector  model=Falling  ic=0  Ts=Ts
  Edge Detector2 : spsEdgeDetectorLib/Edge Detector  model=Rising  ic=0  Ts=Ts
  Edge Detector3 : spsEdgeDetectorLib/Edge Detector  model=Rising  ic=0  Ts=Ts
  Product2 : Product  InputSameDT=on  SaturateOnIntegerOverflow=on  OutDataTypeStr=Inherit: Same as first input
  Relational Operator : RelationalOperator  Operator=>
  Relational Operator2 : RelationalOperator  Operator=<
  Sum5 : Sum  Inputs=+-  InputSameDT=on  SaturateOnIntegerOverflow=on  OutDataTypeStr=Inherit: Same as first input
  Sum6 : Sum  InputSameDT=on  SaturateOnIntegerOverflow=on  OutDataTypeStr=Inherit: Same as first input
  Terminator : Terminator
  Trigonometric Function7 : Trigonometry
  alpha2 : Constant  Value=0
  alpha9 : Constant  Value=pi*Ts
  SqWave : Outport  VectorParamsAs1DForOutWhenUnconnected=off
  Sync + : Outport  Port=2  VectorParamsAs1DForOutWhenUnconnected=off
  Sync - : Outport  Port=3  VectorParamsAs1DForOutWhenUnconnected=off
  wires:
  Data Type Conversion/1 -> Edge Detector/1, Edge Detector1/1, SqWave/1
  Bistable/2 -> Terminator/1
  Edge Detector3/1 -> Bistable/2
  Edge Detector2/1 -> Bistable/1
  Edge Detector1/1 -> Sync -/1
  Edge Detector/1 -> Sync +/1
  Bistable/1 -> Data Type Conversion/1
  alpha9/1 -> Product2/1
  Product2/1 -> Trigonometric Function7/1
  Relational Operator2/1 -> Edge Detector3/1
  Relational Operator/1 -> Edge Detector2/1
  Sum6/1 -> Relational Operator2/2
  Sum5/1 -> Relational Operator/2
  alpha2/1 -> Sum6/1, Sum5/1
  Trigonometric Function7/1 -> Sum6/2, Sum5/2
  Freq/1 -> Product2/2
  sin(wt)/1 -> Relational Operator/1, Relational Operator2/1

== system Hybrid2_article_SVC_stage1/SVC Controller1/Firing Unit/Firing Unit BC/PLL sync on positive peak  ==
  note: Note: -sin( a ) * sin( b ) = 1/2 * cos( a+b ) - 1/2 * cos(a-b)
  note: Discrete 1-phase PLL
  note: Note: PLL synchronized on positive peak of input
  note: Pierre Giroux, Gilbert Sybille
      | Power System Laboratory, IREQ
      | Hydro-Quebec
  V(pu) : Inport
  Constant4 : Constant  Value=2*pi
  Discrete PI Controller : Subsystem  DialogController=POWERSYS.PowerSysDialog  mask(Discrete PI Controller){Kp=Kp, Ki=Ki, Par_Limits=[1.25  0.75]*2*pi*Finit, Init=2*pi*Finit, Ts=Ts}
      mask prompts: Kp "Proportional gain (Kp):"; Ki "Integral gain (Ki):"; Par_Limits "Output limits: [ Upper   Lower ]"; Init "Output initial value:"; Ts "Sample time:"
      mask help: This block implements a discrete PI controller.
      mask init:
      | UpperLimit=Par_Limits(1);
      | LowerLimit=Par_Limits(2);
      | power_initmask();
      mask Help: This block is part of a subset of blocks in the Extras library that does not have documentation associated with it, other than the block mask description.
      mask Display: disp('PI');
  Discrete-Time Integrator : DiscreteIntegrator  InitialCondition=(Phase_Init-90)*pi/180  SampleTime=Ts  ICPrevOutput=DiscIntNeverNeededParam  ICPrevScaledInput=DiscIntNeverNeededParam
  Gain10 : Gain  Gain=1/2/pi  SaturateOnIntegerOverflow=on  OutDataTypeStr=Inherit: Same as input  ParamDataTypeStr=Inherit: Same as input
  Gain12 : Gain  Gain=-1  SaturateOnIntegerOverflow=on  OutDataTypeStr=Inherit: Same as input  ParamDataTypeStr=Inherit: Same as input
  Math Function : Math  Operator=mod  SignedPower=on
  Mean (Variable Frequency)1 : spsMeanVariableFrequencyLib/Mean (Variable Frequency)  Finit=Finit  Fmin=45  Vinit=0  Ts=Ts
  Product1 : Product  InputSameDT=on  SaturateOnIntegerOverflow=on  OutDataTypeStr=Inherit: Same as first input
  Rate Limiter : RateLimiter  RisingSlewLimit=10  FallingSlewLimit=-10  SampleTimeMode=inherited  InitialCondition=Finit
  Second-Order Filter : spsSecondOrderFilterLib/Second-Order Filter  FilterType=Lowpass  Fo=25  Zeta=0.707  Ts=Ts  Initialize=on  Vac_Init="[0 0  Finit]"  Vdc_Init=Finit  PlotResponse=off  FreqRange=[1 500 1]
  Trigonometric Function6 : Trigonometry
  Unit Delay1 : UnitDelay  InitialCondition=Finit  SampleTime=Ts  HasFrameUpgradeWarning=on
      settings: AttributesFormatString=IC = %<InitialCondition>
  Freq : Outport  VectorParamsAs1DForOutWhenUnconnected=off
  wt : Outport  Port=2  VectorParamsAs1DForOutWhenUnconnected=off
  wires:
  Gain12/1 -> Product1/1
  V(pu)/1 -> Gain12/1
  Constant4/1 -> Math Function/2
  Discrete-Time Integrator/1 -> Math Function/1
  Product1/1 -> Mean (Variable Frequency)1/2
  Discrete PI Controller/1(Out) -> Discrete-Time Integrator/1, Gain10/1  "W"
  Gain10/1 -> Rate Limiter/1
  Rate Limiter/1 -> Second-Order Filter/1
  Second-Order Filter/1 -> Unit Delay1/1
  Trigonometric Function6/1 -> Product1/2
  Math Function/1 -> Trigonometric Function6/1, wt/1
  Unit Delay1/1 -> Mean (Variable Frequency)1/1, Freq/1
  Mean (Variable Frequency)1/1 -> Discrete PI Controller/1(Error)
